simulink model "mergedemo"  (Simulink 7.6)
settings: Solver=VariableStepDiscrete  SolverMode=SingleTasking  StartTime=0.0  StopTime=20  MaxStep=.1  RelTol=1e-3  AbsTol=1e-6
libraries: simulink x2
Description:
  | Merging Signals
  | 
  | This interactive demonstration introduces you to the following
  | Simulink(R) concepts.
  | 
  |  * Conditionally executed subsystems
  |  * Logical Operator block
  |  * Boolean signals in Simulink
  |  * Creating alternately enabling subsystems using the Merge block
settings Model: Creator=The MathWorks Inc.  ExtModeTrigMode=oneshot  ExtModeArmWhenConnect=off  ExtModeAutoUpdateStatusClock=off
settings DataIOCC: LimitDataPoints=off
settings OptimizationCC: BlockReduction=off  InlineInvariantSignals=on  InitFltsAndDblsToZero=on  BufferReusableBoundary=off
settings DebuggingCC: SaveWithParameterizedLinksMsg=none  SignalResolutionControl=TryResolveAllWithWarning  SolverPrmCheckMsg=none  MultiTaskDSMMsg=warning  MultiTaskCondExecSysMsg=none  IntegerOverflowMsg=none  BusObjectLabelMismatch=none
settings HardwareCC: TargetUnknown=on
settings RTWCC: IncludeERTFirstTime=on
settings GRTTargetCC: TargetFcnLib=ansi_tfl_tmw.mat

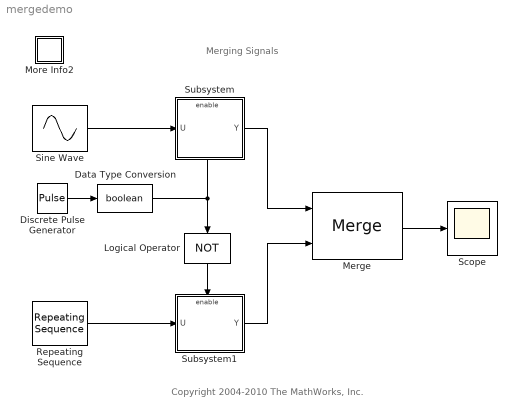
== system mergedemo ==
  note: Merging Signals
  note: Copyright 2004-2010 The MathWorks, Inc.
  Data Type Conversion : DataTypeConversion  OutDataTypeStr=boolean  SaturateOnIntegerOverflow=on  RndMeth=Zero
  Discrete Pulse Generator : DiscretePulseGenerator  SampleTime=5
  Logical Operator : Logic  Operator=NOT  Inputs=1
  Merge : Merge
  More Info2 : Subsystem
      settings: OpenFcn=showdemo(bdroot(gcs))
      mask Display: disp('?')
  Repeating Sequence : simulink/Sources/Repeating Sequence  SystemSampleTime=-1  rep_seq_t=[0 1]  rep_seq_y=[0 2]
  Scope : Scope
      settings: TickLabels=on  TimeRange=20  YMin=-1.5  YMax=2  DataFormat=Array
  Sine Wave : Sin  Frequency=pi  SampleTime=0
  Subsystem : Subsystem  Tag=MergeExample  TreatAsAtomicUnit=on
  Subsystem1 : Subsystem  Tag=MergeExample  TreatAsAtomicUnit=on
  wires:
  Sine Wave/1 -> Subsystem/1(U)
  Subsystem/1(Y) -> Merge/1
  Subsystem1/1(Y) -> Merge/2
  Logical Operator/1 -> Subsystem1/Enable
  Discrete Pulse Generator/1 -> Data Type Conversion/1
  Repeating Sequence/1 -> Subsystem1/1(U)
  Merge/1 -> Scope/1
  Data Type Conversion/1 -> Logical Operator/1, Subsystem/Enable

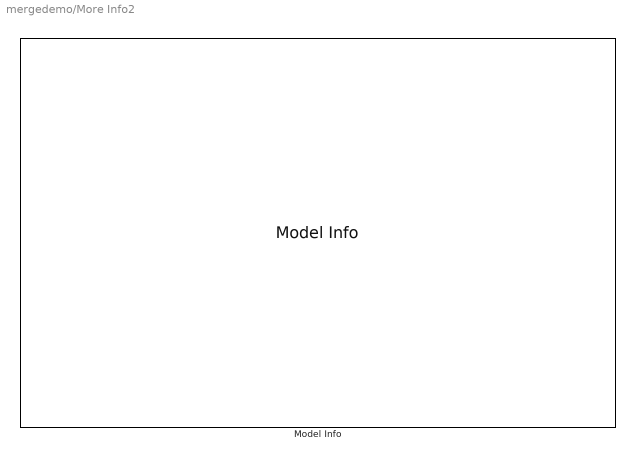
== system mergedemo/More Info2 ==
  Model Info : simulink/Model-Wide Utilities/Model Info  SystemSampleTime=-1  InitialBlockCM=none  BlockCM=None  Frame=on  DisplayStringWithTags=Model Info  HorizontalTextAlignment=Left  LeftAlignmentValue=0.02  SourceBlockDiagram=mergedemo  TagMaxNumber=20

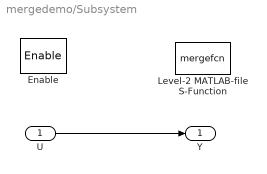
== system mergedemo/Subsystem ==
  U : Inport
  Enable : EnablePort  StatesWhenEnabling=reset
  Level-2 MATLAB-file S-Function : M-S-Function  FunctionName=mergefcn
  Y : Outport
  wires:
  U/1 -> Y/1

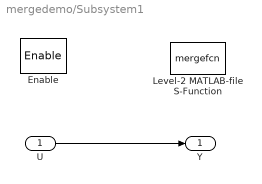
== system mergedemo/Subsystem1 ==
  U : Inport
  Enable : EnablePort  StatesWhenEnabling=reset
  Level-2 MATLAB-file S-Function : M-S-Function  FunctionName=mergefcn
  Y : Outport
  wires:
  U/1 -> Y/1
